simulink model "SD_Lin_cartmodel"  (R2019b)
settings: Solver=ode4  StartTime=0.0  StopTime=stoptime  FixedStep=h  RelTol=1e-6  AbsTol=1e-6  EnableMultiTasking=on
values from neighbouring files (symbols this model uses):
  A = Ab    [mainfile_solution.m]
  B = Bb    [mainfile_solution.m]
  C = Cb    [mainfile_solution.m]
  D = Db    [mainfile_solution.m]
  Kd = place(Ad,Bd,p_z)    [mainfile_solution.m]
  x0_tilde = x0b_tilde    [mainfile_solution.m]
settings Model: Creator=Ale  LastModifiedBy=n9182250
settings SolverCC: AutoScaleAbsTol=off
settings DataIOCC: SaveFormat=Array  SignalLoggingSaveFormat=ModelDataLogs  SaveOutput=off  SaveTime=off  TimeSaveName=t
settings OptimizationCC: ExpressionDepthLimit=2147483647  LifeSpan=inf
settings DebuggingCC: UnderspecifiedInitializationDetection=Classic  MergeDetectMultiDrivingBlocksExec=none  FcnCallInpInsideContextMsg=warning  StateNameClashWarn=warning  SFUnexpectedBacktrackingDiag=warning  SFNoUnconditionalDefaultTransitionDiag=warning  SFExecutionAtInitializationDiag=none  ArithmeticOperatorsInVariantConditions=warning
settings HardwareCC: ProdBitPerPointer=32  ProdBitPerSizeT=32  ProdBitPerPtrDiffT=32  ProdLargestAtomicFloat=None  ProdIntDivRoundTo=Undefined  ProdEndianess=Unspecified  ProdWordSize=32  ProdHWDeviceType=32-bit Generic
settings ModelReferenceCC: PropagateSignalLabelsOutOfModel=off
settings SFSimCC: SimUseLocalCustomCode=off  CustomCodeUndefinedFunction=UseInterfaceOnly
settings RTWCC: RTWUseLocalCustomCode=off
settings CodeAppCC: StateflowObjectComments=on
settings GRTTargetCC: TargetLangStandard=C89/C90 (ANSI)  GeneratePreprocessorConditionals=Disable all  CombineOutputUpdateFcns=off  GRTInterface=on
settings ConfigComp: CovMetricSettings=dw  CovHtmlReporting=on  CovSaveCumulativeToWorkspaceVar=on  CovSaveSingleToWorkspaceVar=on  CovExternalEMLEnable=off

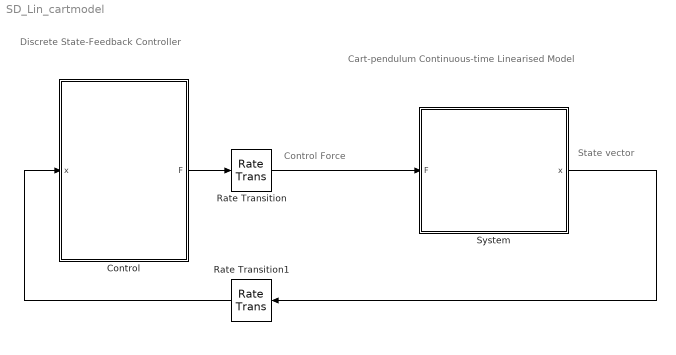
== system SD_Lin_cartmodel ==
  note: Discrete State-Feedback
      | Controller
  note: Control Force
  note: State vector
  note: Cart-pendulum
      | Continuous-time Linearised Model
  Control : Subsystem
  Rate Transition : RateTransition  InitialCondition=-Kd*x0_tilde
  Rate Transition1 : RateTransition  InitialCondition=x0_tilde  OutPortSampleTime=Ts
  System : Subsystem
  wires:
  Control/1(F) -> Rate Transition/1
  Rate Transition/1 -> System/1(F)
  System/1(x) -> Rate Transition1/1
  Rate Transition1/1 -> Control/1(x)

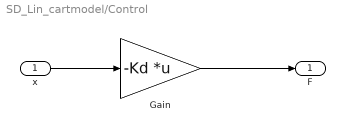
== system SD_Lin_cartmodel/Control ==
  x : Inport
  Gain : Gain  Gain=-Kd  Multiplication=Matrix(K*u)
  F : Outport  VectorParamsAs1DForOutWhenUnconnected=off
  wires:
  x/1 -> Gain/1
  Gain/1 -> F/1

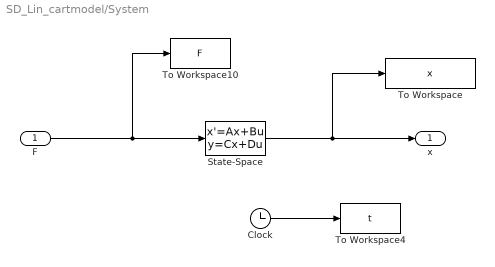
== system SD_Lin_cartmodel/System ==
  F : Inport
  Clock : Clock
  State-Space : StateSpace  A=A  B=B  C=C  D=D  InitialCondition=x0_tilde
  To Workspace : ToWorkspace  VariableName=x  SampleTime=-1
  To Workspace10 : ToWorkspace  VariableName=F  SampleTime=-1
  To Workspace4 : ToWorkspace  VariableName=t  SampleTime=-1
  x : Outport  VectorParamsAs1DForOutWhenUnconnected=off
  wires:
  F/1 -> To Workspace10/1, State-Space/1
  State-Space/1 -> To Workspace/1, x/1
  Clock/1 -> To Workspace4/1
